simulink model "untitled"  (R2015b)
settings: Solver=VariableStepAuto  StartTime=0.0  StopTime=10  RelTol=1e-3
settings Model: Creator=Dmitry  LastModifiedBy=Dmitry

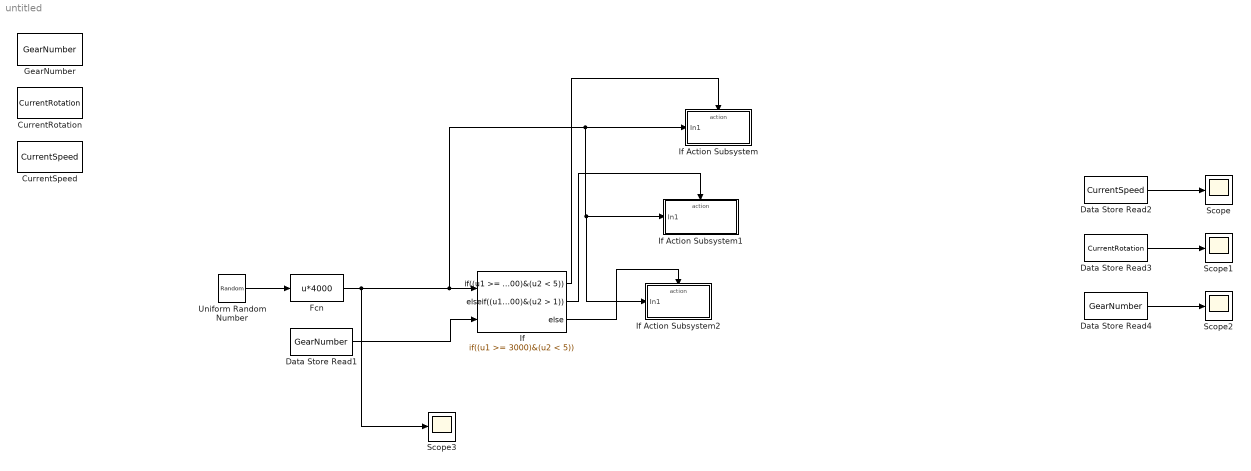
== system untitled ==
  CurrentRotation : DataStoreMemory  DataStoreName=CurrentRotation  ReadBeforeWriteMsg=warning  WriteAfterWriteMsg=warning  WriteAfterReadMsg=warning  InitialValue=800  OutMax=[6000]
  CurrentSpeed : DataStoreMemory  DataStoreName=CurrentSpeed  ReadBeforeWriteMsg=warning  WriteAfterWriteMsg=warning  WriteAfterReadMsg=warning  InitialValue=9.6
  Data Store Read1 : DataStoreRead  DataStoreName=GearNumber
  Data Store Read2 : DataStoreRead  DataStoreName=CurrentSpeed
  Data Store Read3 : DataStoreRead  DataStoreName=CurrentRotation
  Data Store Read4 : DataStoreRead  DataStoreName=GearNumber
  Fcn : Fcn  Expr=u*4000
  GearNumber : DataStoreMemory  DataStoreName=GearNumber  ReadBeforeWriteMsg=warning  WriteAfterWriteMsg=warning  WriteAfterReadMsg=warning  InitialValue=1
  If : If  NumInputs=2  IfExpression=(u1 >= 3000)&(u2 < 5)  ElseIfExpressions=(u1 <= 800)&(u2 > 1)
  If Action Subsystem : Subsystem  TreatAsAtomicUnit=on
  If Action Subsystem1 : Subsystem  TreatAsAtomicUnit=on
  If Action Subsystem2 : Subsystem  TreatAsAtomicUnit=on
  Scope{,1..3} (4 alike) : Scope
  Uniform Random Number : UniformRandomNumber  Minimum=0  Seed=0.5  SampleTime=1
  wires:
  Fcn/1 -> Scope3/1, If Action Subsystem1/1(In1), If Action Subsystem2/1(In1), If Action Subsystem/1(In1), If/1
  Data Store Read1/1 -> If/2
  If/1 -> If Action Subsystem/Action
  Uniform Random Number/1 -> Fcn/1
  Data Store Read2/1 -> Scope/1
  Data Store Read3/1 -> Scope1/1
  Data Store Read4/1 -> Scope2/1
  If/3 -> If Action Subsystem2/Action
  If/2 -> If Action Subsystem1/Action

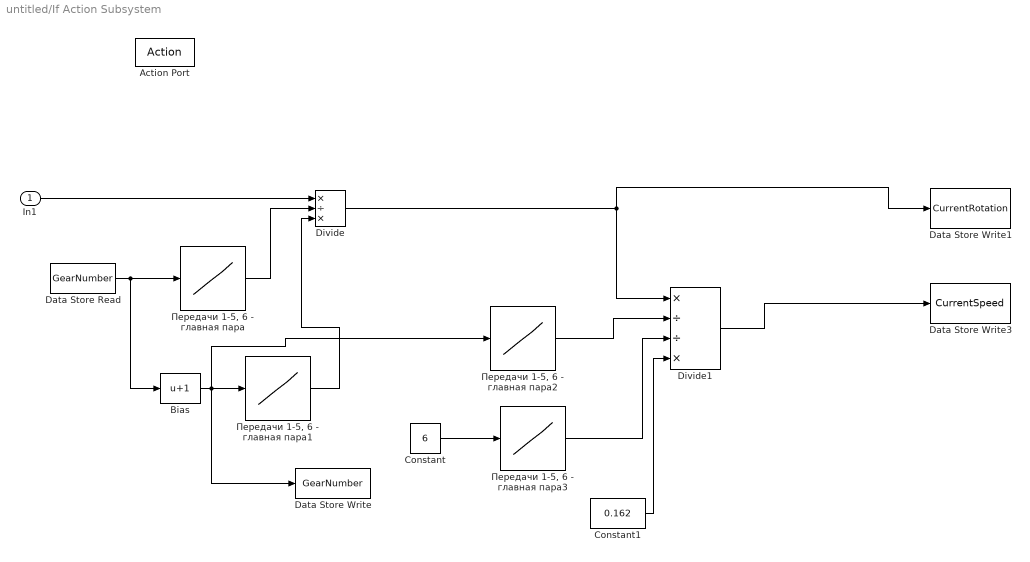
== system untitled/If Action Subsystem ==
  In1 : Inport
  Action Port : ActionPort  PropagateVarSize=During execution  ActionType=then
  Bias : Bias  Bias=1
  Constant : Constant  Value=6
  Constant1 : Constant  Value=0.162  VectorParams1D=off
  Data Store Read : DataStoreRead  DataStoreName=GearNumber
  Data Store Write : DataStoreWrite  DataStoreName=GearNumber
  Data Store Write1 : DataStoreWrite  DataStoreName=CurrentRotation
  Data Store Write3 : DataStoreWrite  DataStoreName=CurrentSpeed
  Divide : Product  Inputs=*/*
  Divide1 : Product  Inputs=*//*
  "Передачи 1-5, 6 - главная пара " : Lookup_n-D  NumberOfTableDimensions=1  BreakpointsForDimension1=[1,2,3,4,5,6]  Table=[3.636;1.95;1.357;0.941;0.784;3.706]  TableDataTypeStr=Inherit: Inherit from 'Table data'  InterpMethod=Flat  DiagnosticForOutOfRangeInput=Error  InternalRulePriority=Speed  RndMeth=Simplest  InputSameDT=on
  "Передачи 1-5, 6 - главная пара1" : Lookup_n-D  NumberOfTableDimensions=1  BreakpointsForDimension1=[1;2;3;4;5;6]  BreakpointsForDimension1DataTypeStr=uint8  Table=[3.636;1.95;1.357;0.941;0.784;3.706]  TableDataTypeStr=double  InterpMethod=Flat  InternalRulePriority=Speed  OutDataTypeStr=double  RndMeth=Simplest  InputSameDT=on
  "Передачи 1-5, 6 - главная пара2" : Lookup_n-D  NumberOfTableDimensions=1  BreakpointsForDimension1=[1;2;3;4;5;6]  BreakpointsForDimension1DataTypeStr=uint8  Table=[3.636;1.95;1.357;0.941;0.784;3.706]  TableDataTypeStr=double  InterpMethod=Flat  InternalRulePriority=Speed  OutDataTypeStr=double  RndMeth=Simplest  InputSameDT=on
  "Передачи 1-5, 6 - главная пара3" : Lookup_n-D  NumberOfTableDimensions=1  BreakpointsForDimension1=[1;2;3;4;5;6]  BreakpointsForDimension1DataTypeStr=uint8  Table=[3.636;1.95;1.357;0.941;0.784;3.706]  TableDataTypeStr=double  InterpMethod=Flat  InternalRulePriority=Speed  OutDataTypeStr=double  RndMeth=Simplest  InputSameDT=on
  wires:
  Data Store Read/1 -> Bias/1, "Передачи 1-5, 6 - главная пара "/1
  Bias/1 -> "Передачи 1-5, 6 - главная пара2"/1, "Передачи 1-5, 6 - главная пара1"/1, Data Store Write/1
  "Передачи 1-5, 6 - главная пара "/1 -> Divide/2
  Divide/1 -> Data Store Write1/1, Divide1/1
  "Передачи 1-5, 6 - главная пара1"/1 -> Divide/3
  In1/1 -> Divide/1
  Constant/1 -> "Передачи 1-5, 6 - главная пара3"/1
  "Передачи 1-5, 6 - главная пара2"/1 -> Divide1/2
  "Передачи 1-5, 6 - главная пара3"/1 -> Divide1/3
  Constant1/1 -> Divide1/4
  Divide1/1 -> Data Store Write3/1

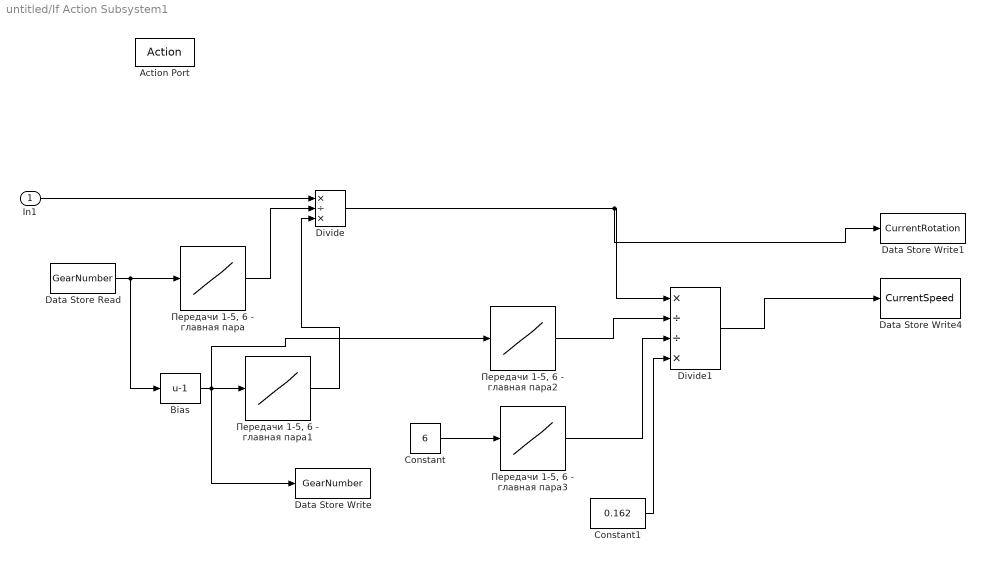
== system untitled/If Action Subsystem1 ==
  In1 : Inport
  Action Port : ActionPort  PropagateVarSize=During execution  ActionType=elseif
  Bias : Bias  Bias=-1
  Constant : Constant  Value=6
  Constant1 : Constant  Value=0.162  VectorParams1D=off
  Data Store Read : DataStoreRead  DataStoreName=GearNumber
  Data Store Write : DataStoreWrite  DataStoreName=GearNumber
  Data Store Write1 : DataStoreWrite  DataStoreName=CurrentRotation
  Data Store Write4 : DataStoreWrite  DataStoreName=CurrentSpeed
  Divide : Product  Inputs=*/*
  Divide1 : Product  Inputs=*//*
  "Передачи 1-5, 6 - главная пара " : Lookup_n-D  NumberOfTableDimensions=1  BreakpointsForDimension1=[1,2,3,4,5,6]  Table=[3.636;1.95;1.357;0.941;0.784;3.706]  TableDataTypeStr=Inherit: Inherit from 'Table data'  InterpMethod=Flat  DiagnosticForOutOfRangeInput=Error  InternalRulePriority=Speed  RndMeth=Simplest  InputSameDT=on
  "Передачи 1-5, 6 - главная пара1" : Lookup_n-D  NumberOfTableDimensions=1  BreakpointsForDimension1=[1;2;3;4;5;6]  BreakpointsForDimension1DataTypeStr=uint8  Table=[3.636;1.95;1.357;0.941;0.784;3.706]  TableDataTypeStr=double  InterpMethod=Flat  InternalRulePriority=Speed  OutDataTypeStr=double  RndMeth=Simplest  InputSameDT=on
  "Передачи 1-5, 6 - главная пара2" : Lookup_n-D  NumberOfTableDimensions=1  BreakpointsForDimension1=[1;2;3;4;5;6]  BreakpointsForDimension1DataTypeStr=uint8  Table=[3.636;1.95;1.357;0.941;0.784;3.706]  TableDataTypeStr=double  InterpMethod=Flat  InternalRulePriority=Speed  OutDataTypeStr=double  RndMeth=Simplest  InputSameDT=on
  "Передачи 1-5, 6 - главная пара3" : Lookup_n-D  NumberOfTableDimensions=1  BreakpointsForDimension1=[1;2;3;4;5;6]  BreakpointsForDimension1DataTypeStr=uint8  Table=[3.636;1.95;1.357;0.941;0.784;3.706]  TableDataTypeStr=double  InterpMethod=Flat  InternalRulePriority=Speed  OutDataTypeStr=double  RndMeth=Simplest  InputSameDT=on
  wires:
  Data Store Read/1 -> Bias/1, "Передачи 1-5, 6 - главная пара "/1
  Bias/1 -> "Передачи 1-5, 6 - главная пара2"/1, "Передачи 1-5, 6 - главная пара1"/1, Data Store Write/1
  "Передачи 1-5, 6 - главная пара "/1 -> Divide/2
  Divide/1 -> Data Store Write1/1, Divide1/1
  "Передачи 1-5, 6 - главная пара1"/1 -> Divide/3
  In1/1 -> Divide/1
  Constant/1 -> "Передачи 1-5, 6 - главная пара3"/1
  "Передачи 1-5, 6 - главная пара2"/1 -> Divide1/2
  "Передачи 1-5, 6 - главная пара3"/1 -> Divide1/3
  Constant1/1 -> Divide1/4
  Divide1/1 -> Data Store Write4/1

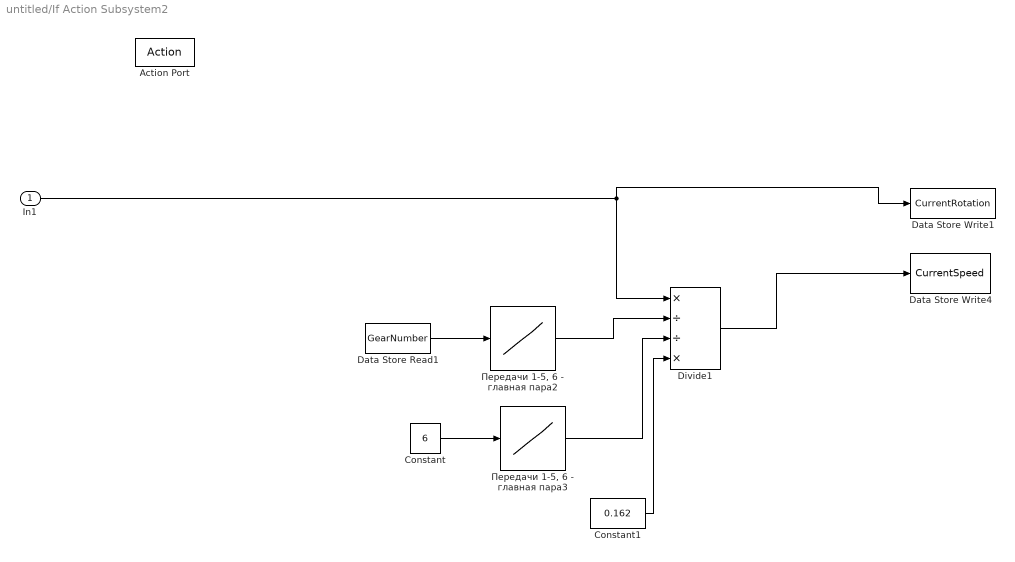
== system untitled/If Action Subsystem2 ==
  In1 : Inport
  Action Port : ActionPort  PropagateVarSize=During execution  ActionType=else
  Constant : Constant  Value=6
  Constant1 : Constant  Value=0.162  VectorParams1D=off
  Data Store Read1 : DataStoreRead  DataStoreName=GearNumber
  Data Store Write1 : DataStoreWrite  DataStoreName=CurrentRotation
  Data Store Write4 : DataStoreWrite  DataStoreName=CurrentSpeed
  Divide1 : Product  Inputs=*//*
  "Передачи 1-5, 6 - главная пара2" : Lookup_n-D  NumberOfTableDimensions=1  BreakpointsForDimension1=[1;2;3;4;5;6]  BreakpointsForDimension1DataTypeStr=uint8  Table=[3.636;1.95;1.357;0.941;0.784;3.706]  TableDataTypeStr=double  InterpMethod=Flat  InternalRulePriority=Speed  OutDataTypeStr=double  RndMeth=Simplest  InputSameDT=on
  "Передачи 1-5, 6 - главная пара3" : Lookup_n-D  NumberOfTableDimensions=1  BreakpointsForDimension1=[1;2;3;4;5;6]  BreakpointsForDimension1DataTypeStr=uint8  Table=[3.636;1.95;1.357;0.941;0.784;3.706]  TableDataTypeStr=double  InterpMethod=Flat  InternalRulePriority=Speed  OutDataTypeStr=double  RndMeth=Simplest  InputSameDT=on
  wires:
  In1/1 -> Divide1/1, Data Store Write1/1
  Data Store Read1/1 -> "Передачи 1-5, 6 - главная пара2"/1
  Constant/1 -> "Передачи 1-5, 6 - главная пара3"/1
  "Передачи 1-5, 6 - главная пара2"/1 -> Divide1/2
  "Передачи 1-5, 6 - главная пара3"/1 -> Divide1/3
  Constant1/1 -> Divide1/4
  Divide1/1 -> Data Store Write4/1
